simulink model "EKF_liuxg"  (R2017a)
settings: Solver=FixedStepAuto  StartTime=0.0  StopTime=13135  FixedStep=1  RelTol=1e-3
undefined symbols (not defined in the file): sigbuilder_block
libraries: dspmtrx3 x2
settings Model: Creator=HP  LastModifiedBy=HP
settings DataIOCC: ReturnWorkspaceOutputs=on
settings DebuggingCC: UnconnectedInputMsg=none  UnconnectedOutputMsg=none  UnconnectedLineMsg=none
settings ModelReferenceCC: EnableRefExpFcnMdlSchedulingChecks=off
settings SFSimCC: SimUseLocalCustomCode=on
settings RTWCC: RTWUseLocalCustomCode=on

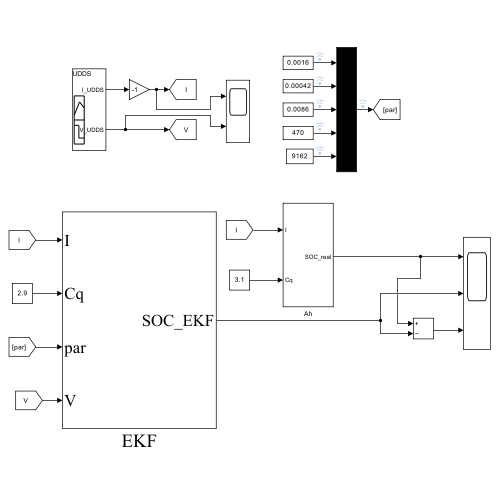
[thumbnail: Simulink's stored preview of the top-level diagram]
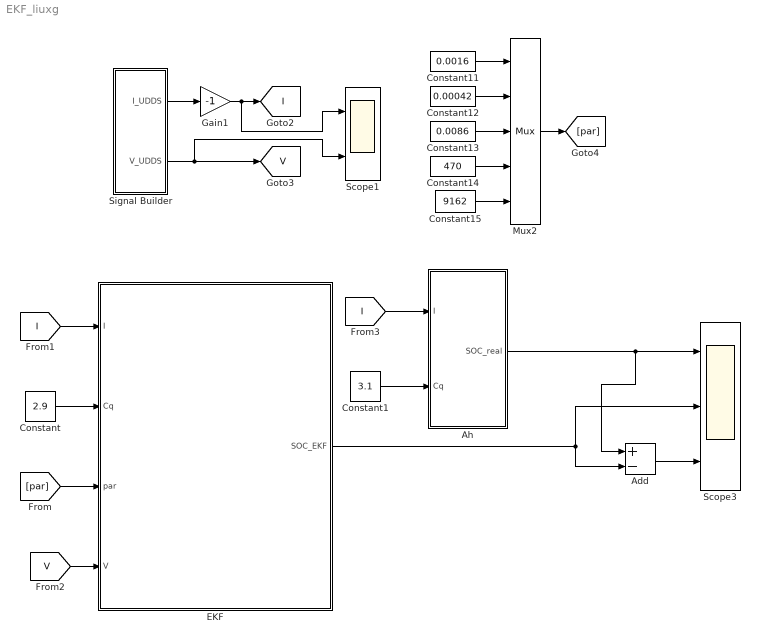
== system EKF_liuxg ==
  Add : Sum  Inputs=+-
  Ah : Subsystem
  Constant : Constant  Value=2.9
  Constant1 : Constant  Value=3.1
  Constant11 : Constant  Value=0.0016
  Constant12 : Constant  Value=0.00042
  Constant13 : Constant  Value=0.0086
  Constant14 : Constant  Value=470
  Constant15 : Constant  Value=9162
  EKF : Subsystem  mask{Q_EKF=[0.0001,0.0001,0.00001], R_EKF=0.01, X0_EKF=[0.8;0;0], P0_EKF=[0.01,0.01,0.01], f_OCV=[-542.328042776627	3066.57848545083	-7520.83333797876	10535.7804287577	-9327.72222618654	5441.66203885271	-2111.60737486106	536.514433511755	-85.4036277861597	8.01612301618486	2.03460000000008]}
      mask prompts: Q_EKF "系统协方差Q"; R_EKF "测量协方差R"; X0_EKF "状态初始值X0"; P0_EKF "估计协方差初始值P0"; f_OCV "开路电压对SOC的函数"
  Gain1 : Gain  Gain=-1
  Mux2 : Mux  Inputs=5
  Scope1 : Scope  NumInputPorts=2
  Scope3 : Scope  NumInputPorts=3
  Signal Builder : Subsystem  Tag=STV Subsys  LoadFcn=sigbuilder_block('load');  StartFcn=sigbuilder_block('start');  StopFcn=sigbuilder_block('stop');  ClipboardFcn=sigbuilder_block('clipboard');  mask(Sigbuilder block){tuvar=[0:10]}
      mask init:
      | if ~strcmp(get_param(bdroot(gcb),'SimulationStatus'),'stopped'),tuvar = sigbuilder_block('maskInit'); end
      settings: CopyFcn=sigbuilder_block('copy');  DeleteFcn=sigbuilder_block('delete');  ModelCloseFcn=sigbuilder_block('modelClose');  PreSaveFcn=sigbuilder_block('preSave');  PauseFcn=sigbuilder_block('pause');  ContinueFcn=sigbuilder_block('continue');  NameChangeFcn=sigbuilder_block('namechange');  OpenFcn=sigbuilder_block('open',[0 63 1141.2 523.8 ]);  CloseFcn=sigbuilder_block('close');
      mask Display: plot(0, 0, 100, 100,[2, 2, 32, 32, 2], [68, 8, 8, 68, 68],[32, 2], [38, 38], [32, 19, 2],[53, 60, 44], [32, 17, 17, 2],[16, 16, 31, 31]);txt = getActiveGroup(gcbh);text(2, 100, txt,'verticalAlignment', 'top');
  tag scope: I=global, V=global
  wires:
  Constant15/1 -> Mux2/5
  Constant11/1 -> Mux2/1
  Constant13/1 -> Mux2/3
  Constant14/1 -> Mux2/4
  Constant12/1 -> Mux2/2
  Mux2/1 -> [par]
  Signal Builder/1(I_UDDS) -> Gain1/1
  Signal Builder/2(V_UDDS) -> [V], Scope1/2
  Gain1/1 -> Scope1/1, [I]
  [par] -> EKF/3(par)
  [I] -> EKF/1(I)
  [V] -> EKF/4(V)
  Constant/1 -> EKF/2(Cq)
  EKF/1(SOC_EKF) -> Scope3/2, Add/2
  [I] -> Ah/1(I)
  Constant1/1 -> Ah/2(Cq)
  Ah/1(SOC_real) -> Add/1, Scope3/1
  Add/1 -> Scope3/3

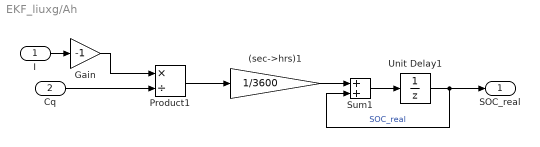
== system EKF_liuxg/Ah ==
  I : Inport
  Cq : Inport  Port=2
  (sec->hrs)1 : Gain  Gain=1/3600  SaturateOnIntegerOverflow=on  OutDataTypeStr=Inherit: Same as input  ParamDataTypeStr=Inherit: Same as input
  Gain : Gain  Gain=-1
  Product1 : Product  Inputs=*/
  Sum1 : Sum
  Unit Delay1 : UnitDelay  InitialCondition=1  SampleTime=-1  HasFrameUpgradeWarning=on
  SOC_real : Outport
  wires:
  I/1 -> Gain/1
  Gain/1 -> Product1/1
  Product1/1 -> (sec->hrs)1/1
  (sec->hrs)1/1 -> Sum1/1
  Unit Delay1/1 -> Sum1/2, SOC_real/1  "SOC_real"
  Sum1/1 -> Unit Delay1/1
  Cq/1 -> Product1/2

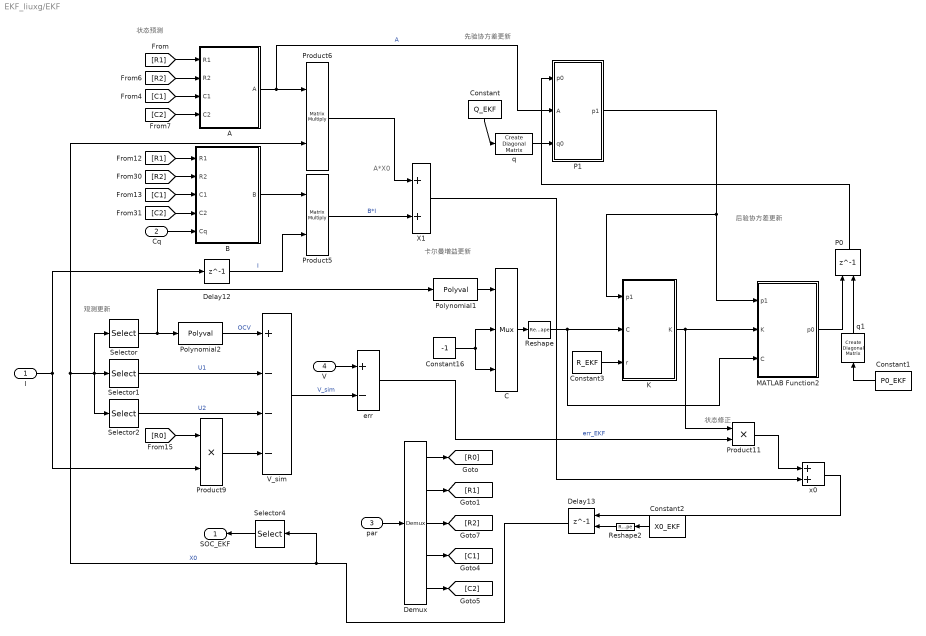
== system EKF_liuxg/EKF ==
  note: 后验协方差更新
  note: 状态修正
  note: 观测更新
  note: 卡尔曼增益更新
  note: 先验协方差更新
  note: 状态预测
  note: A*X0
  I : Inport
  Cq : Inport  Port=2
  par : Inport  Port=3
  V : Inport  Port=4
  A : MATLAB Function  TreatAsAtomicUnit=on
  B : MATLAB Function  TreatAsAtomicUnit=on
  C : Mux  Inputs=3
  Constant : Constant  Value=Q_EKF
  Constant1 : Constant  Value=P0_EKF
  Constant16 : Constant  Value=-1
  Constant2 : Constant  Value=X0_EKF
  Constant3 : Constant  Value=R_EKF
  Delay12 : Delay  DelayLength=1
  Delay13 : Delay  DelayLength=1  InitialConditionSource=Input port  InitialCondition=[.8;0;0]
      settings: InputPortMap=u0,p4
  Demux : Demux  Outputs=5
  K : MATLAB Function  TreatAsAtomicUnit=on
  MATLAB Function2 : MATLAB Function  TreatAsAtomicUnit=on
  P0 : Delay  DelayLength=1  InitialConditionSource=Input port  InitialCondition=0.01*eye(3)
      settings: InputPortMap=u0,p4
  P1 : MATLAB Function  TreatAsAtomicUnit=on
  Polynomial1 : Polyval  Coefs=((length(f_OCV)-1):-1:1).*(f_OCV(1:(length(f_OCV)-1)))
  Polynomial2 : Polyval  Coefs=f_OCV
  Product11 : Product
  Product5 : Product  Multiplication=Matrix(*)
  Product6 : Product  Multiplication=Matrix(*)
  Product9 : Product
  Reshape : Reshape  OutputDimensionality=Customize  OutputDimensions=[1,3]
  Reshape2 : Reshape  OutputDimensionality=Customize  OutputDimensions=[3,1]
  Selector : Selector  InputPortWidth=3  IndexOptions=Index vector (dialog)  Indices=1  OutputSizes=1
  Selector1 : Selector  InputPortWidth=3  IndexOptions=Index vector (dialog)  Indices=2  OutputSizes=1
  Selector2 : Selector  InputPortWidth=3  IndexOptions=Index vector (dialog)  Indices=3  OutputSizes=1
  Selector4 : Selector  InputPortWidth=3  IndexOptions=Index vector (dialog)  Indices=1  OutputSizes=1
  V_sim : Sum  Inputs=+---
  X1 : Sum
  err : Sum  Inputs=+-
  q : dspmtrx3/Create Diagonal Matrix
  q1 : dspmtrx3/Create Diagonal Matrix
  x0 : Sum
  SOC_EKF : Outport
  wires:
  Constant/1 -> q/1
  x0/1 -> Delay13/1
  Demux/1 -> [R0]
  I/1 -> Product9/2, Delay12/1
  V_sim/1 -> err/2  "V_sim"
  K/1(K) -> MATLAB Function2/2(K), Product11/1
  Constant16/1 -> C/2, C/3
  Delay13/1 -> Selector4/1, Product6/2, Selector/1, Selector2/1, Selector1/1  "X0"
  A/1(A) -> P1/2(A), Product6/1  "A"
  Demux/3 -> [R2]
  [R1] -> B/1(R1)
  P1/1(p1) -> K/1(p1), MATLAB Function2/1(p1)
  Delay12/1 -> Product5/2  "I"
  Product6/1 -> X1/1
  Selector2/1 -> V_sim/3  "U2"
  par/1 -> Demux/1
  Polynomial1/1 -> C/1
  P0/1 -> P1/1(p0)
  Selector1/1 -> V_sim/2  "U1"
  Reshape/1 -> MATLAB Function2/3(C), K/2(C)
  Demux/4 -> [C1]
  Constant2/1 -> Reshape2/1
  V/1 -> err/1
  C/1 -> Reshape/1
  Polynomial2/1 -> V_sim/1  "OCV"
  Constant3/1 -> K/3(r)
  Selector/1 -> Polynomial2/1, Polynomial1/1
  Product9/1 -> V_sim/4
  Reshape2/1 -> Delay13/2
  err/1 -> Product11/2  "err_EKF"
  Product5/1 -> X1/2  "B*I"
  Demux/2 -> [R1]
  Cq/1 -> B/5(Cq)
  Demux/5 -> [C2]
  MATLAB Function2/1(p0) -> P0/1
  [C2] -> B/4(C2)
  [R0] -> Product9/1
  q/1 -> P1/3(q0)
  [R1] -> A/1(R1)
  [C2] -> A/4(C2)
  [R2] -> A/2(R2)
  [C1] -> A/3(C1)
  B/1(B) -> Product5/1
  X1/1 -> x0/2
  Product11/1 -> x0/1
  [R2] -> B/2(R2)
  [C1] -> B/3(C1)
  Constant1/1 -> q1/1
  q1/1 -> P0/2
  Selector4/1 -> SOC_EKF/1

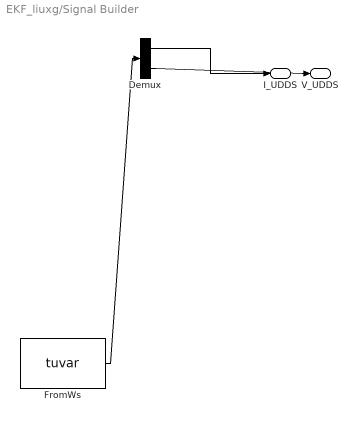
== system EKF_liuxg/Signal Builder ==
  Demux : Demux  Tag=STV Demux  Outputs=2
  FromWs : FromWorkspace  Tag=STV FromWs  VariableName=tuvar
      SigBuilderData=|
      | dataSet.timeRange = [1 13135]
      | dataSet.name = 'UDDS'
      | sbobj.Name = 'Signal Builder'
      | sbobj.Groups.Name = 'UDDS'
      | sbobj.Groups.Signals(1).Name = 'I_UDDS'
      | sbobj.Groups.Signals(1).XData = [1 2 3 4 5 6 7 8 9 10 11 12 ... (13135 elements, 1x13135)]
      | sbobj.Groups.Signals(1).YData = [0 -0.0248 -0.1178 -0.1178 -0.1178 -0.1178 -0.1178 -0.1178 -0.1178 -0.1178 -0.1178 -0.1178 ... (13135 elements, 1x13135)]
      | sbobj.Groups.Signals(2).Name = 'V_UDDS'
      | sbobj.Groups.Signals(2).XData = [1 2 3 4 5 6 7 8 9 10 11 12 ... (13135 elements, 1x13135)]
      | sbobj.Groups.Signals(2).YData = [2.6686 2.6686 2.6683 2.6683 2.6683 2.6677 2.6677 2.6677 2.6677 2.6674 2.6674 2.6674 ... (13135 elements, 1x13135)]
      | sbobj.Groups.TimeRange = [1 9002]
  I_UDDS : Outport  Tag=STV Outport
  V_UDDS : Outport  Tag=STV Outport  Port=2
  wires:
  FromWs/1 -> Demux/1
  Demux/1 -> I_UDDS/1
  Demux/2 -> V_UDDS/1

== matlab function EKF_liuxg/EKF/B ==
  data: R1 input; B output; R2 input; C1 input; C2 input; Cq input
function B = fcn(R1,R2,C1,C2,Cq)
tao1=R1*C1;
tao2=R2*C2;
B=[-1/(3600*Cq);
    R1*(1-exp(-1/tao1));
    R2*(1-exp(-1/tao2))];
end

== matlab function EKF_liuxg/EKF/K ==
  data: p1 input; K output; C input; r input
function K = fcn(p1,C,r)
K=p1*C'/(C*p1*C'+r);
end

== matlab function EKF_liuxg/EKF/P1 ==
  data: p0 input; A input; p1 output; q0 input
function p1= fcn(p0,A,q0)
p1=A*p0*A'+q0;
end

== matlab function EKF_liuxg/EKF/MATLAB Function2 ==
  data: p1 input; p0 output; K input; C input
function p0= fcn(p1,K,C)
p0=p1-K*C*p1;
end

== matlab function EKF_liuxg/EKF/A ==
  data: R1 input; A output; R2 input; C1 input; C2 input
function A = fcn(R1,R2,C1,C2)
tao1=R1*C1;
tao2=R2*C2;
A=[1 0 0;
    0 exp(-1/tao1) 0;
    0 0 exp(-1/tao2)];
end
